simulink model "IEEE30_case"  (R2024b)
settings: Solver=FixedStepAuto  StartTime=0  StopTime=5  FixedStep=1e-7  RelTol=1e-3
values from neighbouring files (symbols this model uses):
  GFL_DFIG_7_C_bus = 0.08    [IEEE30_case_parameters.m]
  GFL_DFIG_7_D_mutual = 2.500000e+3    (= 2500)    [IEEE30_case_parameters.m]
  GFL_DFIG_7_f0 = 60    [IEEE30_case_parameters.m]
  GFL_DFIG_7_gPLLi = 3200    [IEEE30_case_parameters.m]
  GFL_DFIG_7_gPLLp = 650    [IEEE30_case_parameters.m]
  GFL_DFIG_7_H_WT = 0.4    [IEEE30_case_parameters.m]
  GFL_DFIG_7_Hg = 0.8    [IEEE30_case_parameters.m]
  GFL_DFIG_7_Igq_ref = 0    [IEEE30_case_parameters.m]
  GFL_DFIG_7_Ird_ref = 704.45696    [IEEE30_case_parameters.m]
  GFL_DFIG_7_KI_V = -300000    [IEEE30_case_parameters.m]
  GFL_DFIG_7_KP_V = -1000    [IEEE30_case_parameters.m]
  GFL_DFIG_7_Ksh = 1.254300e+4    (= 12543)    [IEEE30_case_parameters.m]
  GFL_DFIG_7_Lg = 0.000483    [IEEE30_case_parameters.m]
  GFL_DFIG_7_Lm_pu = 4    [IEEE30_case_parameters.m]
  GFL_DFIG_7_N = 100    [IEEE30_case_parameters.m]
  GFL_DFIG_7_p = 2    [IEEE30_case_parameters.m]
  GFL_DFIG_7_Pitch = 0    [IEEE30_case_parameters.m]
  GFL_DFIG_7_R = 44    [IEEE30_case_parameters.m]
  GFL_DFIG_7_Rg = 2.000000e-5    (= 2e-05)    [IEEE30_case_parameters.m]
  GFL_DFIG_7_rho = 1.225    [IEEE30_case_parameters.m]
  GFL_DFIG_7_rPLLi = 4500    [IEEE30_case_parameters.m]
  GFL_DFIG_7_rPLLp = 620    [IEEE30_case_parameters.m]
  GFL_DFIG_7_Rs_pu = 0.011    [IEEE30_case_parameters.m]
  GFL_DFIG_7_Sbase = 2.000000e+6    (= 2000000)    [IEEE30_case_parameters.m]
  GFL_DFIG_7_ugq_ref = 0    [IEEE30_case_parameters.m]
  GFL_DFIG_7_usd_ref = 0    [IEEE30_case_parameters.m]
  GFL_DFIG_7_Vbase = 690    [IEEE30_case_parameters.m]
  GFL_DFIG_7_Vdc_ref = 1200    [IEEE30_case_parameters.m]
  GFL_DFIG_7_wind = 12    [IEEE30_case_parameters.m]
  GFL_DFIG_7_wm_ref = 518.184209    [IEEE30_case_parameters.m]
  SG_D_13_D = 0.01056    [IEEE30_case_parameters.m]
  SG_D_13_EnableSaturation = 0    [IEEE30_case_parameters.m]
  SG_D_13_f0 = 60    [IEEE30_case_parameters.m]
  SG_D_13_H = 7.5    [IEEE30_case_parameters.m]
  SG_D_13_K_A = 20    [IEEE30_case_parameters.m]
  SG_D_13_K_E = 1.000000e+1    (= 10)    [IEEE30_case_parameters.m]
  SG_D_13_K_F = 2.363    [IEEE30_case_parameters.m]
  SG_D_13_K_s = 0.5    [IEEE30_case_parameters.m]
  SG_D_13_R_a = 0.001088    [IEEE30_case_parameters.m]
  SG_D_13_S_A = 1    [IEEE30_case_parameters.m]
  SG_D_13_S_B = 0.103    [IEEE30_case_parameters.m]
  SG_D_13_S_N = 10.659857    [IEEE30_case_parameters.m]
  SG_D_13_SpeedPara = 200    [IEEE30_case_parameters.m]
  SG_D_13_T_0 = 0.370163    [IEEE30_case_parameters.m]
  SG_D_13_T_1 = 0.3    [IEEE30_case_parameters.m]
  SG_D_13_T_2 = 0.05    [IEEE30_case_parameters.m]
  SG_D_13_T_3 = 0.02    [IEEE30_case_parameters.m]
  SG_D_13_T_4 = 0.005    [IEEE30_case_parameters.m]
  SG_D_13_T_A = 0.02    [IEEE30_case_parameters.m]
  SG_D_13_T_dd = 8.000000e+0    (= 8)    [IEEE30_case_parameters.m]
  SG_D_13_T_ddd = 0.04    [IEEE30_case_parameters.m]
  SG_D_13_T_E = 0.314    [IEEE30_case_parameters.m]
  SG_D_13_T_F = 0.35    [IEEE30_case_parameters.m]
  SG_D_13_T_qd = 0.8    [IEEE30_case_parameters.m]
  SG_D_13_T_qdd = 0.02    [IEEE30_case_parameters.m]
  SG_D_13_T_speed = 0.1    [IEEE30_case_parameters.m]
  SG_D_13_T_w = 0.5    [IEEE30_case_parameters.m]
  SG_D_13_V_ref = 1.696619    [IEEE30_case_parameters.m]
  SG_D_13_w_ref = 376.991118    [IEEE30_case_parameters.m]
  SG_D_13_x_d = 1.9    [IEEE30_case_parameters.m]
  SG_D_13_x_dd = 0.302    [IEEE30_case_parameters.m]
  SG_D_13_x_ddd = 0.204    [IEEE30_case_parameters.m]
  SG_D_13_x_l = 0.05    [IEEE30_case_parameters.m]
  SG_D_13_x_q = 1.3    [IEEE30_case_parameters.m]
  SG_D_13_x_qd = 0.5    [IEEE30_case_parameters.m]
  SG_D_13_x_qdd = 0.3    [IEEE30_case_parameters.m]
  SG_D_1_D = 0.01056    [IEEE30_case_parameters.m]
  SG_D_1_EnableSaturation = 0    [IEEE30_case_parameters.m]
  SG_D_1_f0 = 60    [IEEE30_case_parameters.m]
  SG_D_1_H = 7.5    [IEEE30_case_parameters.m]
  SG_D_1_K_A = 20    [IEEE30_case_parameters.m]
  SG_D_1_K_E = 1.000000e+1    (= 10)    [IEEE30_case_parameters.m]
  SG_D_1_K_F = 2.363    [IEEE30_case_parameters.m]
  SG_D_1_K_s = 0.5    [IEEE30_case_parameters.m]
  SG_D_1_R_a = 0.001088    [IEEE30_case_parameters.m]
  SG_D_1_S_A = 1    [IEEE30_case_parameters.m]
  SG_D_1_S_B = 0.103    [IEEE30_case_parameters.m]
  SG_D_1_S_N = 10.659857    [IEEE30_case_parameters.m]
  SG_D_1_SpeedPara = 200    [IEEE30_case_parameters.m]
  SG_D_1_T_0 = 0.259812    [IEEE30_case_parameters.m]
  SG_D_1_T_1 = 0.3    [IEEE30_case_parameters.m]
  SG_D_1_T_2 = 0.05    [IEEE30_case_parameters.m]
  SG_D_1_T_3 = 0.02    [IEEE30_case_parameters.m]
  SG_D_1_T_4 = 0.005    [IEEE30_case_parameters.m]
  SG_D_1_T_A = 0.02    [IEEE30_case_parameters.m]
  SG_D_1_T_dd = 8.000000e+0    (= 8)    [IEEE30_case_parameters.m]
  SG_D_1_T_ddd = 0.04    [IEEE30_case_parameters.m]
  SG_D_1_T_E = 0.314    [IEEE30_case_parameters.m]
  SG_D_1_T_F = 0.35    [IEEE30_case_parameters.m]
  SG_D_1_T_qd = 0.8    [IEEE30_case_parameters.m]
  SG_D_1_T_qdd = 0.02    [IEEE30_case_parameters.m]
  SG_D_1_T_speed = 0.1    [IEEE30_case_parameters.m]
  SG_D_1_T_w = 0.5    [IEEE30_case_parameters.m]
  SG_D_1_V_ref = 1.544107    [IEEE30_case_parameters.m]
  SG_D_1_w_ref = 376.991118    [IEEE30_case_parameters.m]
  SG_D_1_x_d = 1.9    [IEEE30_case_parameters.m]
  SG_D_1_x_dd = 0.302    [IEEE30_case_parameters.m]
  SG_D_1_x_ddd = 0.204    [IEEE30_case_parameters.m]
  SG_D_1_x_l = 0.05    [IEEE30_case_parameters.m]
  SG_D_1_x_q = 1.3    [IEEE30_case_parameters.m]
  SG_D_1_x_qd = 0.5    [IEEE30_case_parameters.m]
  SG_D_1_x_qdd = 0.3    [IEEE30_case_parameters.m]
  SG_D_22_D = 0.01056    [IEEE30_case_parameters.m]
  SG_D_22_EnableSaturation = 0    [IEEE30_case_parameters.m]
  SG_D_22_f0 = 60    [IEEE30_case_parameters.m]
  SG_D_22_H = 7.5    [IEEE30_case_parameters.m]
  SG_D_22_K_A = 20    [IEEE30_case_parameters.m]
  SG_D_22_K_E = 1.000000e+1    (= 10)    [IEEE30_case_parameters.m]
  SG_D_22_K_F = 2.363    [IEEE30_case_parameters.m]
  SG_D_22_K_s = 0.5    [IEEE30_case_parameters.m]
  SG_D_22_R_a = 0.001088    [IEEE30_case_parameters.m]
  SG_D_22_S_A = 1    [IEEE30_case_parameters.m]
  SG_D_22_S_B = 0.103    [IEEE30_case_parameters.m]
  SG_D_22_S_N = 10.659857    [IEEE30_case_parameters.m]
  SG_D_22_SpeedPara = 200    [IEEE30_case_parameters.m]
  SG_D_22_T_0 = 0.216121    [IEEE30_case_parameters.m]
  SG_D_22_T_1 = 0.3    [IEEE30_case_parameters.m]
  SG_D_22_T_2 = 0.05    [IEEE30_case_parameters.m]
  SG_D_22_T_3 = 0.02    [IEEE30_case_parameters.m]
  SG_D_22_T_4 = 0.005    [IEEE30_case_parameters.m]
  ... (+126 more)
(part 25 of 27)

== system IEEE30_case/SG_D_23/d_w_SG_D_23_block ==
  note: d_w_SG_D_23 in IEEE30_case
      | $\frac{2\,\pi \,T_{m,\mathrm{SG},D,23}\,f_{0}-D\,\left(w_{\mathrm{SG},D,23}-2\,\pi \,f_{0}\right)+2\,\pi \,f_{0}\,\left(\frac{\psi _{d,\mathrm{SG},D,23}\,\left(\psi _{q,\mathrm{SG},D,23}+\frac{\psi _{\mathrm{gq},\mathrm{SG},D,23}\,\left(x_{l}-x_{\mathrm{qdd}}\right)}{x_{l}-x_{\mathrm{qd}}}+\frac{\psi _{\mathrm{kq},\mathrm{SG},D,23}\,\left(x_{\mathrm{qd}}-x_{\mathrm{qdd}}\right)}{x_{l}-x_{\mathrm{qd}}}\right)}{x_{\mathrm{qdd}}}+\frac{\psi _{q,\mathrm{SG},D,23}\,\left(\frac{\psi _{\mathrm{1d},\mathrm{SG},D,23}\,\left(x_{\mathrm{dd}}-x_{\mathrm{ddd}}\right)}{x_{\mathrm{dd}}-x_{l}}-\psi _{d,\mathrm{SG},D,23}+\frac{\psi _{\mathrm{fd},\mathrm{SG},D,23}\,\left(x_{\mathrm{ddd}}-x_{l}\right)}{x_{\mathrm{dd}}-x_{l}}\right)}{x_{\mathrm{ddd}}}\right)}{2\,H}$
      | Automatically generated on 2025-11-01 18:37:27 .
  State_w_SG_D_23_a9c86 : Inport
  State_T_m_SG_D_23_67386 : Inport  Port=2
  State_psi_d_SG_D_23_cd292 : Inport  Port=3
  State_psi_gq_SG_D_23_30ca6 : Inport  Port=4
  State_psi_kq_SG_D_23_85da1 : Inport  Port=5
  State_psi_q_SG_D_23_ea802 : Inport  Port=6
  State_psi_q_SG_D_23_f4578 : Inport  Port=7
  State_psi_1d_SG_D_23_250d1 : Inport  Port=8
  State_psi_d_SG_D_23_77cdf : Inport  Port=9
  State_psi_fd_SG_D_23_fba26 : Inport  Port=10
  Add_34a9a : Sum
  Add_60312 : Sum
  Add_766b7 : Sum
  Add_877ab : Sum
  Add_a2dd3 : Sum
  Add_bf21f : Sum
  Add_cbb42 : Sum
  Add_ce37c : Sum
  Constant_-1_0529d : Constant  Value=-1
  Constant_-1_0665a : Constant  Value=-1
  Constant_-1_1274e : Constant  Value=-1
  Constant_-1_ae622 : Constant  Value=-1
  Constant_-1_bb572 : Constant  Value=-1
  Constant_-1_d880a : Constant  Value=-1
  Constant_-2.0_7e7ab : Constant  Value=-2.0
  Constant_2.0_0eeaf : Constant  Value=2.0
  Constant_2.0_8133d : Constant  Value=2.0
  Constant_2.0_86630 : Constant  Value=2.0
  Constant_D_d8423 : Constant  Value=D
  Constant_H_9e85c : Constant  Value=H
  Constant_f0_0164f : Constant  Value=f0
  Constant_f0_37545 : Constant  Value=f0
  Constant_f0_adf10 : Constant  Value=f0
  Constant_pi_89cee : Constant  Value=pi
  Constant_pi_ad3cb : Constant  Value=pi
  Constant_pi_f19cc : Constant  Value=pi
  Constant_x_dd_2dfc0 : Constant  Value=x_dd
  Constant_x_dd_49240 : Constant  Value=x_dd
  Constant_x_dd_d4555 : Constant  Value=x_dd
  Constant_x_ddd_5b4e5 : Constant  Value=x_ddd
  Constant_x_ddd_79b99 : Constant  Value=x_ddd
  Constant_x_ddd_80fee : Constant  Value=x_ddd
  Constant_x_l_03679 : Constant  Value=x_l
  Constant_x_l_34a4f : Constant  Value=x_l
  Constant_x_l_64425 : Constant  Value=x_l
  Constant_x_l_756be : Constant  Value=x_l
  Constant_x_l_91cbf : Constant  Value=x_l
  Constant_x_l_c7781 : Constant  Value=x_l
  Constant_x_qd_92bf4 : Constant  Value=x_qd
  Constant_x_qd_a2a78 : Constant  Value=x_qd
  Constant_x_qd_dda99 : Constant  Value=x_qd
  Constant_x_qdd_3c8ce : Constant  Value=x_qdd
  Constant_x_qdd_41b30 : Constant  Value=x_qdd
  Constant_x_qdd_81d75 : Constant  Value=x_qdd
  Divide_438bc : Product  Inputs=*/
  Divide_5c9e7 : Product  Inputs=*/
  Divide_64d37 : Product  Inputs=*/
  Divide_9ddc5 : Product  Inputs=*/
  Divide_c63d1 : Product  Inputs=*/
  Divide_dc8c0 : Product  Inputs=*/
  Divide_ea4bc : Product  Inputs=*/
  Product_024c1 : Product
  Product_072d4 : Product
  Product_1a3ea : Product
  Product_24bca : Product
  Product_392d6 : Product
  Product_3abdb : Product
  Product_4016c : Product
  Product_514ef : Product
  Product_55414 : Product
  Product_579b0 : Product
  Product_5df71 : Product
  Product_70ed9 : Product
  Product_75340 : Product
  Product_78ecf : Product
  Product_88dc9 : Product
  Product_8ee02 : Product
  Product_b37c8 : Product
  Product_c9e22 : Product
  Product_d29a1 : Product
  Product_eba4f : Product
  Product_ec235 : Product
  Product_f29ae : Product
  Subtract_30638 : Sum  Inputs=+-
  Subtract_5bb39 : Sum  Inputs=+-
  Subtract_a0565 : Sum  Inputs=+-
  Subtract_cf16a : Sum  Inputs=+-
  Subtract_cf1ab : Sum  Inputs=+-
  Subtract_d4472 : Sum  Inputs=+-
  Subtract_e17ae : Sum  Inputs=+-
  Subtract_f98fa : Sum  Inputs=+-
  Blockout_d_w_SG_D_23_057d1 : Outport
  wires:
  Constant_x_qdd_3c8ce/1 -> Add_877ab/2
  Constant_-1_0529d/1 -> Product_eba4f/1
  Product_eba4f/1 -> Add_877ab/1
  Constant_x_l_03679/1 -> Product_eba4f/2
  Product_78ecf/1 -> Add_a2dd3/1
  Constant_-1_bb572/1 -> Product_78ecf/1
  Subtract_cf1ab/1 -> Product_024c1/2
  Constant_x_qd_dda99/1 -> Subtract_cf1ab/1
  Constant_x_l_756be/1 -> Product_78ecf/2
  Constant_D_d8423/1 -> Product_d29a1/2
  Constant_x_qdd_41b30/1 -> Subtract_cf1ab/2
  Product_392d6/1 -> Add_cbb42/1
  Constant_-1_ae622/1 -> Product_392d6/1
  Constant_x_ddd_80fee/1 -> Subtract_cf16a/2
  Constant_-1_d880a/1 -> Product_d29a1/1
  Subtract_30638/1 -> Divide_438bc/2
  Constant_x_l_64425/1 -> Product_392d6/2
  Constant_-1_0665a/1 -> Product_5df71/1
  State_psi_1d_SG_D_23_250d1/1 -> Product_5df71/2
  State_psi_q_SG_D_23_ea802/1 -> Add_ce37c/2
  Constant_x_dd_d4555/1 -> Subtract_cf16a/1
  Constant_x_l_c7781/1 -> Subtract_a0565/2
  Product_579b0/1 -> Divide_ea4bc/1
  State_psi_gq_SG_D_23_30ca6/1 -> Product_579b0/1
  Add_877ab/1 -> Product_579b0/2
  Constant_x_qd_a2a78/1 -> Add_a2dd3/2
  Product_024c1/1 -> Divide_64d37/1
  State_psi_kq_SG_D_23_85da1/1 -> Product_024c1/1
  Subtract_cf16a/1 -> Product_1a3ea/2
  Constant_x_qd_92bf4/1 -> Add_cbb42/2
  Product_5df71/1 -> Product_1a3ea/1
  Constant_x_dd_2dfc0/1 -> Subtract_30638/1
  State_w_SG_D_23_a9c86/1 -> Add_766b7/2
  Product_ec235/1 -> Product_c9e22/1
  Constant_x_l_91cbf/1 -> Subtract_30638/2
  Constant_-1_1274e/1 -> Product_ec235/1
  Subtract_d4472/1 -> Product_8ee02/2
  Constant_x_ddd_5b4e5/1 -> Subtract_d4472/1
  Constant_x_l_34a4f/1 -> Subtract_d4472/2
  Constant_-2.0_7e7ab/1 -> Product_70ed9/1
  Add_a2dd3/1 -> Divide_ea4bc/2
  Add_cbb42/1 -> Divide_64d37/2
  Product_1a3ea/1 -> Divide_438bc/1
  Constant_2.0_8133d/1 -> Product_4016c/1
  Product_8ee02/1 -> Divide_5c9e7/1
  State_psi_fd_SG_D_23_fba26/1 -> Product_8ee02/1
  Subtract_a0565/1 -> Divide_5c9e7/2
  Constant_x_dd_49240/1 -> Subtract_a0565/1
  Divide_ea4bc/1 -> Subtract_5bb39/1
  Divide_64d37/1 -> Subtract_5bb39/2
  Divide_438bc/1 -> Add_60312/1
  State_psi_d_SG_D_23_77cdf/1 -> Add_60312/2
  Constant_pi_ad3cb/1 -> Product_70ed9/2
  State_psi_d_SG_D_23_cd292/1 -> Product_ec235/2
  Subtract_5bb39/1 -> Add_ce37c/1
  Add_60312/1 -> Subtract_e17ae/1
  Divide_5c9e7/1 -> Subtract_e17ae/2
  Product_70ed9/1 -> Product_514ef/1
  Constant_f0_0164f/1 -> Product_514ef/2
  Constant_pi_f19cc/1 -> Product_4016c/2
  Add_ce37c/1 -> Product_c9e22/2
  State_psi_q_SG_D_23_f4578/1 -> Product_b37c8/1
  Subtract_e17ae/1 -> Product_b37c8/2
  Product_514ef/1 -> Add_766b7/1
  Product_4016c/1 -> Product_75340/1
  State_T_m_SG_D_23_67386/1 -> Product_75340/2
  Constant_2.0_86630/1 -> Product_88dc9/1
  Constant_pi_89cee/1 -> Product_88dc9/2
  Product_c9e22/1 -> Divide_9ddc5/1
  Constant_x_qdd_81d75/1 -> Divide_9ddc5/2
  Product_b37c8/1 -> Divide_c63d1/1
  Constant_x_ddd_79b99/1 -> Divide_c63d1/2
  Product_d29a1/1 -> Product_072d4/1
  Add_766b7/1 -> Product_072d4/2
  Product_75340/1 -> Product_24bca/1
  Constant_f0_37545/1 -> Product_24bca/2
  Product_88dc9/1 -> Product_55414/1
  Constant_f0_adf10/1 -> Product_55414/2
  Divide_9ddc5/1 -> Add_bf21f/1
  Divide_c63d1/1 -> Add_bf21f/2
  Product_072d4/1 -> Add_34a9a/1
  Product_24bca/1 -> Add_34a9a/2
  Product_55414/1 -> Product_f29ae/1
  Add_bf21f/1 -> Product_f29ae/2
  Add_34a9a/1 -> Subtract_f98fa/1
  Product_f29ae/1 -> Subtract_f98fa/2
  Constant_2.0_0eeaf/1 -> Product_3abdb/1
  Constant_H_9e85c/1 -> Product_3abdb/2
  Subtract_f98fa/1 -> Divide_dc8c0/1
  Product_3abdb/1 -> Divide_dc8c0/2
  Divide_dc8c0/1 -> Blockout_d_w_SG_D_23_057d1/1

== system IEEE30_case/SG_D_23/i_d_SG_D_23_block ==
  note: i_d_SG_D_23 in IEEE30_case
      | $\frac{\sin\left(\theta _{\mathrm{SG},D,23}\right)\,\left(\frac{\psi _{\mathrm{1d},\mathrm{SG},D,23}\,\left(x_{\mathrm{dd}}-x_{\mathrm{ddd}}\right)}{x_{\mathrm{dd}}-x_{l}}-\psi _{d,\mathrm{SG},D,23}+\frac{\psi _{\mathrm{fd},\mathrm{SG},D,23}\,\left(x_{\mathrm{ddd}}-x_{l}\right)}{x_{\mathrm{dd}}-x_{l}}\right)}{x_{\mathrm{ddd}}}-\frac{\cos\left(\theta _{\mathrm{SG},D,23}\right)\,\left(\psi _{q,\mathrm{SG},D,23}+\frac{\psi _{\mathrm{gq},\mathrm{SG},D,23}\,\left(x_{l}-x_{\mathrm{qdd}}\right)}{x_{l}-x_{\mathrm{qd}}}+\frac{\psi _{\mathrm{kq},\mathrm{SG},D,23}\,\left(x_{\mathrm{qd}}-x_{\mathrm{qdd}}\right)}{x_{l}-x_{\mathrm{qd}}}\right)}{x_{\mathrm{qdd}}}$
      | Automatically generated on 2025-11-01 18:37:45 .
  State_psi_gq_SG_D_23_8a76e : Inport
  State_psi_kq_SG_D_23_a0ec4 : Inport  Port=2
  State_psi_q_SG_D_23_9f429 : Inport  Port=3
  State_theta_SG_D_23_46601 : Inport  Port=4
  State_psi_1d_SG_D_23_7111a : Inport  Port=5
  State_psi_d_SG_D_23_079bd : Inport  Port=6
  State_psi_fd_SG_D_23_8232a : Inport  Port=7
  State_theta_SG_D_23_15384 : Inport  Port=8
  Add_99617 : Sum
  Add_de10d : Sum
  Add_ed57c : Sum
  Add_ee6b8 : Sum
  Add_f683e : Sum
  Constant_-1_312cc : Constant  Value=-1
  Constant_-1_34ed3 : Constant  Value=-1
  Constant_-1_50e02 : Constant  Value=-1
  Constant_-1_7dce9 : Constant  Value=-1
  Constant_-1_936aa : Constant  Value=-1
  Constant_x_dd_20a3c : Constant  Value=x_dd
  Constant_x_dd_90625 : Constant  Value=x_dd
  Constant_x_dd_ca463 : Constant  Value=x_dd
  Constant_x_ddd_32f6c : Constant  Value=x_ddd
  Constant_x_ddd_7f849 : Constant  Value=x_ddd
  Constant_x_ddd_81b41 : Constant  Value=x_ddd
  Constant_x_l_22fb0 : Constant  Value=x_l
  Constant_x_l_3e953 : Constant  Value=x_l
  Constant_x_l_a1a1b : Constant  Value=x_l
  Constant_x_l_adba4 : Constant  Value=x_l
  Constant_x_l_c18b0 : Constant  Value=x_l
  Constant_x_l_db77a : Constant  Value=x_l
  Constant_x_qd_42c43 : Constant  Value=x_qd
  Constant_x_qd_7ef8d : Constant  Value=x_qd
  Constant_x_qd_b32fb : Constant  Value=x_qd
  Constant_x_qdd_7adc2 : Constant  Value=x_qdd
  Constant_x_qdd_837f5 : Constant  Value=x_qdd
  Constant_x_qdd_d77aa : Constant  Value=x_qdd
  Divide_259dc : Product  Inputs=*/
  Divide_31088 : Product  Inputs=*/
  Divide_79f4f : Product  Inputs=*/
  Divide_8d708 : Product  Inputs=*/
  Divide_f1559 : Product  Inputs=*/
  Divide_f7422 : Product  Inputs=*/
  MathFunc_cos_3d1b4 : Trigonometry  Operator=cos
  MathFunc_sin_1f2ca : Trigonometry
  Product_08031 : Product
  Product_2355a : Product
  Product_27067 : Product
  Product_418f8 : Product
  Product_6afa1 : Product
  Product_76679 : Product
  Product_7783e : Product
  Product_addf1 : Product
  Product_dc801 : Product
  Product_e0db2 : Product
  Product_f83ce : Product
  Subtract_0158c : Sum  Inputs=+-
  Subtract_04828 : Sum  Inputs=+-
  Subtract_19bce : Sum  Inputs=+-
  Subtract_2e06c : Sum  Inputs=+-
  Subtract_400c8 : Sum  Inputs=+-
  Subtract_86aa4 : Sum  Inputs=+-
  Subtract_87269 : Sum  Inputs=+-
  Subtract_fd2e5 : Sum  Inputs=+-
  Blockout_i_d_SG_D_23_e5d44 : Outport
  wires:
  Product_addf1/1 -> Divide_f1559/1
  Constant_-1_312cc/1 -> Product_dc801/1
  Constant_x_qdd_d77aa/1 -> Add_f683e/2
  Divide_79f4f/1 -> Subtract_19bce/2
  Constant_-1_50e02/1 -> Product_f83ce/1
  Product_7783e/1 -> Divide_79f4f/1
  State_psi_fd_SG_D_23_8232a/1 -> Product_7783e/1
  Constant_x_l_22fb0/1 -> Product_f83ce/2
  Product_2355a/1 -> Product_76679/1
  Product_6afa1/1 -> Divide_8d708/1
  Constant_x_qdd_7adc2/1 -> Subtract_87269/2
  Divide_f7422/1 -> Subtract_04828/1
  Product_f83ce/1 -> Add_f683e/1
  Constant_-1_7dce9/1 -> Product_e0db2/1
  MathFunc_cos_3d1b4/1 -> Product_08031/2
  State_theta_SG_D_23_46601/1 -> MathFunc_cos_3d1b4/1
  Constant_x_l_adba4/1 -> Product_e0db2/2
  Constant_x_qd_b32fb/1 -> Subtract_87269/1
  Subtract_19bce/1 -> Product_addf1/1
  Add_ee6b8/1 -> Divide_8d708/2
  Constant_x_l_db77a/1 -> Product_dc801/2
  Add_de10d/1 -> Divide_259dc/2
  State_psi_gq_SG_D_23_8a76e/1 -> Product_6afa1/1
  Add_f683e/1 -> Product_6afa1/2
  Product_e0db2/1 -> Add_ee6b8/1
  Constant_x_qd_7ef8d/1 -> Add_ee6b8/2
  Constant_-1_936aa/1 -> Product_2355a/1
  State_psi_kq_SG_D_23_a0ec4/1 -> Product_27067/1
  Subtract_87269/1 -> Product_27067/2
  Product_dc801/1 -> Add_de10d/1
  Constant_x_qd_42c43/1 -> Add_de10d/2
  State_psi_1d_SG_D_23_7111a/1 -> Product_2355a/2
  Constant_x_ddd_7f849/1 -> Divide_f1559/2
  Constant_x_dd_ca463/1 -> Subtract_fd2e5/1
  Constant_x_ddd_81b41/1 -> Subtract_fd2e5/2
  Product_27067/1 -> Divide_259dc/1
  Add_99617/1 -> Product_418f8/2
  Subtract_fd2e5/1 -> Product_76679/2
  Constant_x_dd_20a3c/1 -> Subtract_2e06c/1
  Constant_x_l_a1a1b/1 -> Subtract_2e06c/2
  Subtract_400c8/1 -> Product_7783e/2
  Constant_x_ddd_32f6c/1 -> Subtract_400c8/1
  Constant_x_l_3e953/1 -> Subtract_400c8/2
  Divide_8d708/1 -> Subtract_0158c/1
  Divide_259dc/1 -> Subtract_0158c/2
  Product_08031/1 -> Divide_f7422/1
  Product_76679/1 -> Divide_31088/1
  Subtract_2e06c/1 -> Divide_31088/2
  Subtract_86aa4/1 -> Divide_79f4f/2
  Constant_x_dd_90625/1 -> Subtract_86aa4/1
  Constant_x_l_c18b0/1 -> Subtract_86aa4/2
  Subtract_0158c/1 -> Add_99617/1
  State_psi_q_SG_D_23_9f429/1 -> Add_99617/2
  Divide_31088/1 -> Add_ed57c/1
  State_psi_d_SG_D_23_079bd/1 -> Add_ed57c/2
  Constant_-1_34ed3/1 -> Product_418f8/1
  Add_ed57c/1 -> Subtract_19bce/1
  MathFunc_sin_1f2ca/1 -> Product_addf1/2
  State_theta_SG_D_23_15384/1 -> MathFunc_sin_1f2ca/1
  Subtract_04828/1 -> Blockout_i_d_SG_D_23_e5d44/1
  Constant_x_qdd_837f5/1 -> Divide_f7422/2
  Product_418f8/1 -> Product_08031/1
  Divide_f1559/1 -> Subtract_04828/2

== system IEEE30_case/SG_D_23/i_q_SG_D_23_block ==
  note: i_q_SG_D_23 in IEEE30_case
      | $-\frac{\sin\left(\theta _{\mathrm{SG},D,23}\right)\,\left(\psi _{q,\mathrm{SG},D,23}+\frac{\psi _{\mathrm{gq},\mathrm{SG},D,23}\,\left(x_{l}-x_{\mathrm{qdd}}\right)}{x_{l}-x_{\mathrm{qd}}}+\frac{\psi _{\mathrm{kq},\mathrm{SG},D,23}\,\left(x_{\mathrm{qd}}-x_{\mathrm{qdd}}\right)}{x_{l}-x_{\mathrm{qd}}}\right)}{x_{\mathrm{qdd}}}-\frac{\cos\left(\theta _{\mathrm{SG},D,23}\right)\,\left(\frac{\psi _{\mathrm{1d},\mathrm{SG},D,23}\,\left(x_{\mathrm{dd}}-x_{\mathrm{ddd}}\right)}{x_{\mathrm{dd}}-x_{l}}-\psi _{d,\mathrm{SG},D,23}+\frac{\psi _{\mathrm{fd},\mathrm{SG},D,23}\,\left(x_{\mathrm{ddd}}-x_{l}\right)}{x_{\mathrm{dd}}-x_{l}}\right)}{x_{\mathrm{ddd}}}$
      | Automatically generated on 2025-11-01 18:37:50 .
  State_psi_gq_SG_D_23_3b4c4 : Inport
  State_psi_kq_SG_D_23_d1d5c : Inport  Port=2
  State_psi_q_SG_D_23_c45ba : Inport  Port=3
  State_theta_SG_D_23_c31a3 : Inport  Port=4
  State_psi_1d_SG_D_23_19122 : Inport  Port=5
  State_psi_d_SG_D_23_577bb : Inport  Port=6
  State_psi_fd_SG_D_23_b9ece : Inport  Port=7
  State_theta_SG_D_23_c16ba : Inport  Port=8
  Add_40d8d : Sum
  Add_4ae2a : Sum
  Add_573c3 : Sum
  Add_6cdcb : Sum
  Add_cfaac : Sum
  Add_f2645 : Sum
  Constant_-1_58374 : Constant  Value=-1
  Constant_-1_5d3a0 : Constant  Value=-1
  Constant_-1_c6427 : Constant  Value=-1
  Constant_-1_c999f : Constant  Value=-1
  Constant_-1_e8bcc : Constant  Value=-1
  Constant_x_dd_a0767 : Constant  Value=x_dd
  Constant_x_dd_aad58 : Constant  Value=x_dd
  Constant_x_dd_b9b12 : Constant  Value=x_dd
  Constant_x_ddd_3afe5 : Constant  Value=x_ddd
  Constant_x_ddd_65fae : Constant  Value=x_ddd
  Constant_x_ddd_885b5 : Constant  Value=x_ddd
  Constant_x_l_20736 : Constant  Value=x_l
  Constant_x_l_2a9d6 : Constant  Value=x_l
  Constant_x_l_3a9f1 : Constant  Value=x_l
  Constant_x_l_72430 : Constant  Value=x_l
  Constant_x_l_c5284 : Constant  Value=x_l
  Constant_x_l_d083f : Constant  Value=x_l
  Constant_x_qd_355aa : Constant  Value=x_qd
  Constant_x_qd_52434 : Constant  Value=x_qd
  Constant_x_qd_d7bb4 : Constant  Value=x_qd
  Constant_x_qdd_01ebd : Constant  Value=x_qdd
  Constant_x_qdd_aa134 : Constant  Value=x_qdd
  Constant_x_qdd_f67ba : Constant  Value=x_qdd
  Divide_13908 : Product  Inputs=*/
  Divide_13ab8 : Product  Inputs=*/
  Divide_2d93d : Product  Inputs=*/
  Divide_30293 : Product  Inputs=*/
  Divide_59a04 : Product  Inputs=*/
  Divide_8c936 : Product  Inputs=*/
  MathFunc_cos_790f2 : Trigonometry  Operator=cos
  MathFunc_sin_f0776 : Trigonometry
  Product_0bb89 : Product
  Product_2ae1e : Product
  Product_6a635 : Product
  Product_76692 : Product
  Product_98dff : Product
  Product_b23ed : Product
  Product_c9e90 : Product
  Product_e90a6 : Product
  Product_f576e : Product
  Product_f7fec : Product
  Product_fcf6b : Product
  Subtract_0c11d : Sum  Inputs=+-
  Subtract_640c1 : Sum  Inputs=+-
  Subtract_94cc8 : Sum  Inputs=+-
  Subtract_ba012 : Sum  Inputs=+-
  Subtract_c2950 : Sum  Inputs=+-
  Subtract_d2e13 : Sum  Inputs=+-
  Subtract_e8b1e : Sum  Inputs=+-
  Blockout_i_q_SG_D_23_6ad1e : Outport
  wires:
  Constant_x_ddd_65fae/1 -> Subtract_e8b1e/2
  Constant_x_l_20736/1 -> Product_f576e/2
  Constant_-1_58374/1 -> Product_f576e/1
  Product_f576e/1 -> Add_4ae2a/1
  Product_76692/1 -> Product_98dff/1
  Constant_-1_c999f/1 -> Product_76692/1
  Constant_x_qdd_01ebd/1 -> Subtract_c2950/2
  Constant_x_qdd_f67ba/1 -> Add_4ae2a/2
  Constant_x_qdd_aa134/1 -> Divide_2d93d/2
  Product_b23ed/1 -> Add_6cdcb/1
  Constant_-1_5d3a0/1 -> Product_b23ed/1
  Add_cfaac/1 -> Blockout_i_q_SG_D_23_6ad1e/1
  Add_40d8d/1 -> Product_6a635/2
  Product_c9e90/1 -> Divide_13908/1
  Subtract_c2950/1 -> Product_e90a6/2
  Constant_x_qd_355aa/1 -> Subtract_c2950/1
  Constant_x_l_d083f/1 -> Product_b23ed/2
  Product_2ae1e/1 -> Divide_2d93d/1
  Product_fcf6b/1 -> Add_f2645/1
  Constant_-1_c6427/1 -> Product_fcf6b/1
  Constant_x_l_2a9d6/1 -> Product_fcf6b/2
  MathFunc_cos_790f2/1 -> Product_0bb89/2
  State_theta_SG_D_23_c16ba/1 -> MathFunc_cos_790f2/1
  State_psi_1d_SG_D_23_19122/1 -> Product_76692/2
  State_psi_gq_SG_D_23_3b4c4/1 -> Product_c9e90/1
  Constant_-1_e8bcc/1 -> Product_6a635/1
  Add_4ae2a/1 -> Product_c9e90/2
  MathFunc_sin_f0776/1 -> Product_2ae1e/2
  Constant_x_qd_d7bb4/1 -> Add_6cdcb/2
  Product_e90a6/1 -> Divide_13ab8/1
  State_psi_kq_SG_D_23_d1d5c/1 -> Product_e90a6/1
  Constant_x_qd_52434/1 -> Add_f2645/2
  Constant_x_l_72430/1 -> Subtract_d2e13/2
  Subtract_e8b1e/1 -> Product_98dff/2
  Constant_x_dd_a0767/1 -> Subtract_e8b1e/1
  Add_6cdcb/1 -> Divide_13908/2
  Add_f2645/1 -> Divide_13ab8/2
  Subtract_0c11d/1 -> Divide_59a04/2
  Constant_x_dd_aad58/1 -> Subtract_0c11d/1
  Constant_x_l_c5284/1 -> Subtract_0c11d/2
  Subtract_640c1/1 -> Product_f7fec/2
  Constant_x_ddd_3afe5/1 -> Subtract_640c1/1
  Constant_x_l_3a9f1/1 -> Subtract_640c1/2
  Divide_13908/1 -> Subtract_ba012/1
  Divide_13ab8/1 -> Subtract_ba012/2
  Product_98dff/1 -> Divide_59a04/1
  Product_f7fec/1 -> Divide_8c936/1
  State_psi_fd_SG_D_23_b9ece/1 -> Product_f7fec/1
  Subtract_d2e13/1 -> Divide_8c936/2
  Constant_x_dd_b9b12/1 -> Subtract_d2e13/1
  Subtract_ba012/1 -> Add_40d8d/1
  State_psi_q_SG_D_23_c45ba/1 -> Add_40d8d/2
  Divide_59a04/1 -> Add_573c3/1
  State_psi_d_SG_D_23_577bb/1 -> Add_573c3/2
  State_theta_SG_D_23_c31a3/1 -> MathFunc_sin_f0776/1
  Product_6a635/1 -> Product_2ae1e/1
  Add_573c3/1 -> Subtract_94cc8/1
  Divide_8c936/1 -> Subtract_94cc8/2
  Subtract_94cc8/1 -> Product_0bb89/1
  Product_0bb89/1 -> Divide_30293/1
  Constant_x_ddd_885b5/1 -> Divide_30293/2
  Divide_2d93d/1 -> Add_cfaac/1
  Divide_30293/1 -> Add_cfaac/2

== system IEEE30_case/SG_D_23/theta_SG_D_23_out_block ==
  note: theta_SG_D_23_out in IEEE30_case
      | $\theta _{\mathrm{SG},D,23}$
      | Automatically generated on 2025-11-01 18:37:55 .
  State_theta_SG_D_23_9d978 : Inport
  Blockout_theta_SG_D_23_out_f3dde : Outport
  wires:
  State_theta_SG_D_23_9d978/1 -> Blockout_theta_SG_D_23_out_f3dde/1

== system IEEE30_case/SG_D_23/w_SG_D_23_out_block ==
  note: w_SG_D_23_out in IEEE30_case
      | $w_{\mathrm{SG},D,23}$
      | Automatically generated on 2025-11-01 18:37:55 .
  State_w_SG_D_23_a1e59 : Inport
  Blockout_w_SG_D_23_out_6070a : Outport
  wires:
  State_w_SG_D_23_a1e59/1 -> Blockout_w_SG_D_23_out_6070a/1

== system IEEE30_case/SG_D_27/T_e_SG_D_27_block ==
  note: T_e_SG_D_27 in IEEE30_case
      | $-\frac{\psi _{d,\mathrm{SG},D,27}\,\left(\psi _{q,\mathrm{SG},D,27}+\frac{\psi _{\mathrm{gq},\mathrm{SG},D,27}\,\left(x_{l}-x_{\mathrm{qdd}}\right)}{x_{l}-x_{\mathrm{qd}}}+\frac{\psi _{\mathrm{kq},\mathrm{SG},D,27}\,\left(x_{\mathrm{qd}}-x_{\mathrm{qdd}}\right)}{x_{l}-x_{\mathrm{qd}}}\right)}{x_{\mathrm{qdd}}}-\frac{\psi _{q,\mathrm{SG},D,27}\,\left(\frac{\psi _{\mathrm{1d},\mathrm{SG},D,27}\,\left(x_{\mathrm{dd}}-x_{\mathrm{ddd}}\right)}{x_{\mathrm{dd}}-x_{l}}-\psi _{d,\mathrm{SG},D,27}+\frac{\psi _{\mathrm{fd},\mathrm{SG},D,27}\,\left(x_{\mathrm{ddd}}-x_{l}\right)}{x_{\mathrm{dd}}-x_{l}}\right)}{x_{\mathrm{ddd}}}$
      | Automatically generated on 2025-11-01 18:39:03 .
  State_psi_d_SG_D_27_aae51 : Inport
  State_psi_gq_SG_D_27_2222e : Inport  Port=2
  State_psi_kq_SG_D_27_9e25d : Inport  Port=3
  State_psi_q_SG_D_27_c3716 : Inport  Port=4
  State_psi_q_SG_D_27_f2155 : Inport  Port=5
  State_psi_1d_SG_D_27_3beb4 : Inport  Port=6
  State_psi_d_SG_D_27_1e6e0 : Inport  Port=7
  State_psi_fd_SG_D_27_93998 : Inport  Port=8
  Add_58dd4 : Sum
  Add_62b21 : Sum
  Add_6e466 : Sum
  Add_899d1 : Sum
  Add_bf566 : Sum
  Add_cc99a : Sum
  Constant_-1_0339b : Constant  Value=-1
  Constant_-1_76629 : Constant  Value=-1
  Constant_-1_a29db : Constant  Value=-1
  Constant_-1_aebb2 : Constant  Value=-1
  Constant_-1_e217e : Constant  Value=-1
  Constant_x_dd_1da9f : Constant  Value=x_dd
  Constant_x_dd_4bd6a : Constant  Value=x_dd
  Constant_x_dd_a2584 : Constant  Value=x_dd
  Constant_x_ddd_0b1a3 : Constant  Value=x_ddd
  Constant_x_ddd_d560c : Constant  Value=x_ddd
  Constant_x_ddd_e9a7e : Constant  Value=x_ddd
  Constant_x_l_0705f : Constant  Value=x_l
  Constant_x_l_1c38b : Constant  Value=x_l
  Constant_x_l_37715 : Constant  Value=x_l
  Constant_x_l_4b2a4 : Constant  Value=x_l
  Constant_x_l_7000a : Constant  Value=x_l
  Constant_x_l_7b0ba : Constant  Value=x_l
  Constant_x_qd_1bbcc : Constant  Value=x_qd
  Constant_x_qd_51226 : Constant  Value=x_qd
  Constant_x_qd_613e8 : Constant  Value=x_qd
  Constant_x_qdd_0cc21 : Constant  Value=x_qdd
  Constant_x_qdd_249d0 : Constant  Value=x_qdd
  Constant_x_qdd_3834a : Constant  Value=x_qdd
  Divide_62fff : Product  Inputs=*/
  Divide_676ea : Product  Inputs=*/
  Divide_b3eff : Product  Inputs=*/
  Divide_b4cfc : Product  Inputs=*/
  Divide_c55f5 : Product  Inputs=*/
  Divide_dca8c : Product  Inputs=*/
  Product_27d11 : Product
  Product_371ec : Product
  Product_676e4 : Product
  Product_86347 : Product
  Product_8cf2a : Product
  Product_a3725 : Product
  Product_aa5a8 : Product
  Product_b0103 : Product
  Product_b28be : Product
  Product_c1c10 : Product
  Product_cc939 : Product
  Subtract_0b899 : Sum  Inputs=+-
  Subtract_12b2d : Sum  Inputs=+-
  Subtract_5e278 : Sum  Inputs=+-
  Subtract_96f38 : Sum  Inputs=+-
  Subtract_c8542 : Sum  Inputs=+-
  Subtract_e2867 : Sum  Inputs=+-
  Subtract_ee4c3 : Sum  Inputs=+-
  Blockout_T_e_SG_D_27_0afee : Outport
  wires:
  Divide_62fff/1 -> Add_cc99a/1
  Product_cc939/1 -> Divide_676ea/1
  Constant_-1_e217e/1 -> Product_86347/1
  Constant_x_qdd_0cc21/1 -> Add_bf566/2
  Subtract_96f38/1 -> Product_c1c10/2
  Subtract_5e278/1 -> Product_cc939/2
  Constant_x_l_0705f/1 -> Product_86347/2
  State_psi_1d_SG_D_27_3beb4/1 -> Product_371ec/2
  Product_86347/1 -> Add_bf566/1
  Add_6e466/1 -> Blockout_T_e_SG_D_27_0afee/1
  Product_c1c10/1 -> Divide_dca8c/1
  Constant_-1_76629/1 -> Product_a3725/1
  Add_cc99a/1 -> Subtract_96f38/1
  Constant_x_qd_1bbcc/1 -> Subtract_5e278/1
  Product_a3725/1 -> Add_899d1/1
  Constant_x_l_4b2a4/1 -> Product_a3725/2
  Product_b0103/1 -> Product_8cf2a/1
  Constant_x_qdd_249d0/1 -> Subtract_5e278/2
  Constant_-1_a29db/1 -> Product_aa5a8/1
  Constant_x_l_7b0ba/1 -> Product_aa5a8/2
  Constant_x_ddd_e9a7e/1 -> Divide_dca8c/2
  Constant_-1_aebb2/1 -> Product_371ec/1
  Constant_x_dd_1da9f/1 -> Subtract_c8542/1
  Constant_x_ddd_0b1a3/1 -> Subtract_c8542/2
  State_psi_gq_SG_D_27_2222e/1 -> Product_b28be/1
  Subtract_12b2d/1 -> Divide_b4cfc/2
  Add_bf566/1 -> Product_b28be/2
  Constant_x_qd_51226/1 -> Add_899d1/2
  Product_27d11/1 -> Divide_62fff/1
  State_psi_kq_SG_D_27_9e25d/1 -> Product_cc939/1
  Product_aa5a8/1 -> Add_62b21/1
  Constant_x_qd_613e8/1 -> Add_62b21/2
  Constant_x_l_37715/1 -> Subtract_12b2d/2
  Product_371ec/1 -> Product_27d11/1
  Subtract_c8542/1 -> Product_27d11/2
  Constant_x_dd_4bd6a/1 -> Subtract_e2867/1
  Constant_-1_0339b/1 -> Product_b0103/1
  Constant_x_l_1c38b/1 -> Subtract_e2867/2
  Constant_x_ddd_d560c/1 -> Subtract_0b899/1
  Divide_b3eff/1 -> Add_6e466/1
  Constant_x_l_7000a/1 -> Subtract_0b899/2
  State_psi_q_SG_D_27_f2155/1 -> Product_c1c10/1
  Product_b28be/1 -> Divide_c55f5/1
  Add_899d1/1 -> Divide_c55f5/2
  Add_62b21/1 -> Divide_676ea/2
  Subtract_e2867/1 -> Divide_62fff/2
  Add_58dd4/1 -> Product_8cf2a/2
  State_psi_fd_SG_D_27_93998/1 -> Product_676e4/1
  Subtract_0b899/1 -> Product_676e4/2
  Constant_x_dd_a2584/1 -> Subtract_12b2d/1
  Divide_c55f5/1 -> Subtract_ee4c3/1
  Divide_dca8c/1 -> Add_6e466/2
  Divide_676ea/1 -> Subtract_ee4c3/2
  State_psi_d_SG_D_27_1e6e0/1 -> Add_cc99a/2
  Product_676e4/1 -> Divide_b4cfc/1
  Product_8cf2a/1 -> Divide_b3eff/1
  State_psi_d_SG_D_27_aae51/1 -> Product_b0103/2
  Subtract_ee4c3/1 -> Add_58dd4/1
  State_psi_q_SG_D_27_c3716/1 -> Add_58dd4/2
  Divide_b4cfc/1 -> Subtract_96f38/2
  Constant_x_qdd_3834a/1 -> Divide_b3eff/2

== system IEEE30_case/SG_D_27/d_E_fd_SG_D_27_block ==
  note: d_E_fd_SG_D_27 in IEEE30_case
      | $\frac{V_{f,\mathrm{SG},D,27}-E_{\mathrm{fd},\mathrm{SG},D,27}\,K_{E}}{T_{E}}$
      | Automatically generated on 2025-11-01 18:38:46 .
  State_E_fd_SG_D_27_823cb : Inport
  State_V_f_SG_D_27_0da35 : Inport  Port=2
  Add_48682 : Sum
  Constant_-1_b8de2 : Constant  Value=-1
  Constant_K_E_0e495 : Constant  Value=K_E
  Constant_T_E_fb76b : Constant  Value=T_E
  Divide_654ca : Product  Inputs=*/
  Product_5b916 : Product
  Product_f51cd : Product
  Blockout_d_E_fd_SG_D_27_b9ef8 : Outport
  wires:
  State_E_fd_SG_D_27_823cb/1 -> Product_5b916/2
  Constant_-1_b8de2/1 -> Product_5b916/1
  Constant_K_E_0e495/1 -> Product_f51cd/2
  Product_5b916/1 -> Product_f51cd/1
  Add_48682/1 -> Divide_654ca/1
  Divide_654ca/1 -> Blockout_d_E_fd_SG_D_27_b9ef8/1
  Product_f51cd/1 -> Add_48682/1
  State_V_f_SG_D_27_0da35/1 -> Add_48682/2
  Constant_T_E_fb76b/1 -> Divide_654ca/2

== system IEEE30_case/SG_D_27/d_Px_1_SG_D_27_block ==
  note: d_Px_1_SG_D_27 in IEEE30_case
      | $\frac{w_{\mathrm{SG},D,27}-2\,\pi \,f_{0}}{T_{w}}-\frac{\mathrm{Px}_{1,\mathrm{SG},D,27}}{T_{w}}$
      | Automatically generated on 2025-11-01 18:38:47 .
  State_Px_1_SG_D_27_e0716 : Inport
  State_w_SG_D_27_cf173 : Inport  Port=2
  Add_22452 : Sum
  Add_afb5d : Sum
  Constant_-1_262bf : Constant  Value=-1
  Constant_-2.0_7f85f : Constant  Value=-2.0
  Constant_T_w_1847e : Constant  Value=T_w
  Constant_T_w_34261 : Constant  Value=T_w
  Constant_f0_c26b3 : Constant  Value=f0
  Constant_pi_44e21 : Constant  Value=pi
  Divide_7c605 : Product  Inputs=*/
  Divide_a225a : Product  Inputs=*/
  Product_103b8 : Product
  Product_12144 : Product
  Product_362eb : Product
  Blockout_d_Px_1_SG_D_27_439b8 : Outport
  wires:
  Constant_-2.0_7f85f/1 -> Product_362eb/1
  Product_103b8/1 -> Add_22452/1
  Constant_pi_44e21/1 -> Product_362eb/2
  Constant_f0_c26b3/1 -> Product_103b8/2
  Product_362eb/1 -> Product_103b8/1
  State_w_SG_D_27_cf173/1 -> Add_22452/2
  Constant_-1_262bf/1 -> Product_12144/1
  State_Px_1_SG_D_27_e0716/1 -> Product_12144/2
  Product_12144/1 -> Divide_7c605/1
  Constant_T_w_34261/1 -> Divide_7c605/2
  Add_22452/1 -> Divide_a225a/1
  Constant_T_w_1847e/1 -> Divide_a225a/2
  Divide_7c605/1 -> Add_afb5d/1
  Divide_a225a/1 -> Add_afb5d/2
  Add_afb5d/1 -> Blockout_d_Px_1_SG_D_27_439b8/1

== system IEEE30_case/SG_D_27/d_Px_2_SG_D_27_block ==
  note: d_Px_2_SG_D_27 in IEEE30_case
      | $\frac{\mathrm{Px}_{1,\mathrm{SG},D,27}-T_{2}\,\left(\frac{\mathrm{Px}_{1,\mathrm{SG},D,27}}{T_{w}}-\frac{w_{\mathrm{SG},D,27}-2\,\pi \,f_{0}}{T_{w}}\right)}{T_{1}}-\frac{\mathrm{Px}_{2,\mathrm{SG},D,27}}{T_{1}}$
      | Automatically generated on 2025-11-01 18:38:49 .
  State_Px_2_SG_D_27_373db : Inport
  State_Px_1_SG_D_27_13dd5 : Inport  Port=2
  State_Px_1_SG_D_27_849c9 : Inport  Port=3
  State_w_SG_D_27_5c50a : Inport  Port=4
  Add_46263 : Sum
  Add_47a2b : Sum
  Add_59103 : Sum
  Add_94a02 : Sum
  Constant_-1_08b4f : Constant  Value=-1
  Constant_-1_ffc91 : Constant  Value=-1
  Constant_-2.0_6cb4a : Constant  Value=-2.0
  Constant_T_1_09a42 : Constant  Value=T_1
  Constant_T_1_7d634 : Constant  Value=T_1
  Constant_T_2_00f19 : Constant  Value=T_2
  Constant_T_w_9b1ed : Constant  Value=T_w
  Constant_T_w_fb965 : Constant  Value=T_w
  Constant_f0_06efd : Constant  Value=f0
  Constant_pi_67fa7 : Constant  Value=pi
  Divide_631f6 : Product  Inputs=*/
  Divide_84317 : Product  Inputs=*/
  Divide_cc441 : Product  Inputs=*/
  Divide_f707a : Product  Inputs=*/
  Product_14717 : Product
  Product_26973 : Product
  Product_64866 : Product
  Product_bd34f : Product
  Product_cc03e : Product
  Blockout_d_Px_2_SG_D_27_55afa : Outport
  wires:
  Divide_631f6/1 -> Add_47a2b/1
  State_Px_1_SG_D_27_849c9/1 -> Product_bd34f/2
  Constant_f0_06efd/1 -> Product_cc03e/2
  Constant_-2.0_6cb4a/1 -> Product_26973/1
  Product_26973/1 -> Product_cc03e/1
  Product_cc03e/1 -> Add_46263/1
  Constant_pi_67fa7/1 -> Product_26973/2
  Product_bd34f/1 -> Divide_631f6/1
  Constant_-1_08b4f/1 -> Product_bd34f/1
  Divide_84317/1 -> Add_94a02/1
  State_w_SG_D_27_5c50a/1 -> Add_46263/2
  Product_64866/1 -> Add_59103/2
  Constant_T_2_00f19/1 -> Product_64866/1
  Constant_T_w_fb965/1 -> Divide_631f6/2
  Add_46263/1 -> Divide_f707a/1
  Constant_T_w_9b1ed/1 -> Divide_f707a/2
  Divide_f707a/1 -> Add_47a2b/2
  Add_47a2b/1 -> Product_64866/2
  Constant_-1_ffc91/1 -> Product_14717/1
  State_Px_2_SG_D_27_373db/1 -> Product_14717/2
  Add_59103/1 -> Divide_cc441/1
  State_Px_1_SG_D_27_13dd5/1 -> Add_59103/1
  Product_14717/1 -> Divide_84317/1
  Constant_T_1_09a42/1 -> Divide_84317/2
  Constant_T_1_7d634/1 -> Divide_cc441/2
  Divide_cc441/1 -> Add_94a02/2
  Add_94a02/1 -> Blockout_d_Px_2_SG_D_27_55afa/1

== system IEEE30_case/SG_D_27/d_Px_3_SG_D_27_block ==
  note: d_Px_3_SG_D_27 in IEEE30_case
      | $\frac{\mathrm{Px}_{2,\mathrm{SG},D,27}+T_{4}\,\left(\frac{\mathrm{Px}_{1,\mathrm{SG},D,27}-T_{2}\,\left(\frac{\mathrm{Px}_{1,\mathrm{SG},D,27}}{T_{w}}-\frac{w_{\mathrm{SG},D,27}-2\,\pi \,f_{0}}{T_{w}}\right)}{T_{1}}-\frac{\mathrm{Px}_{2,\mathrm{SG},D,27}}{T_{1}}\right)}{T_{3}}-\frac{\mathrm{Px}_{3,\mathrm{SG},D,27}}{T_{3}}$
      | Automatically generated on 2025-11-01 18:38:51 .
  State_Px_3_SG_D_27_7eb86 : Inport
  State_Px_2_SG_D_27_7e14b : Inport  Port=2
  State_Px_2_SG_D_27_a8fab : Inport  Port=3
  State_Px_1_SG_D_27_bbb95 : Inport  Port=4
  State_Px_1_SG_D_27_e5cc3 : Inport  Port=5
  State_w_SG_D_27_62987 : Inport  Port=6
  Add_51e20 : Sum
  Add_a4816 : Sum
  Add_b8d7b : Sum
  Add_b9876 : Sum
  Add_f9525 : Sum
  Add_fe742 : Sum
  Constant_-1_1cd6b : Constant  Value=-1
  Constant_-1_a4f86 : Constant  Value=-1
  Constant_-1_ce658 : Constant  Value=-1
  Constant_-2.0_efe86 : Constant  Value=-2.0
  Constant_T_1_24092 : Constant  Value=T_1
  Constant_T_1_95641 : Constant  Value=T_1
  Constant_T_2_d9632 : Constant  Value=T_2
  Constant_T_3_4372a : Constant  Value=T_3
  Constant_T_3_6a972 : Constant  Value=T_3
  Constant_T_4_5ce1d : Constant  Value=T_4
  Constant_T_w_5790c : Constant  Value=T_w
  Constant_T_w_d4fd1 : Constant  Value=T_w
  Constant_f0_24778 : Constant  Value=f0
  Constant_pi_ac239 : Constant  Value=pi
  Divide_17362 : Product  Inputs=*/
  Divide_22c96 : Product  Inputs=*/
  Divide_87250 : Product  Inputs=*/
  Divide_95976 : Product  Inputs=*/
  Divide_e705a : Product  Inputs=*/
  Divide_ea44b : Product  Inputs=*/
  Product_60ff9 : Product
  Product_6fd5f : Product
  Product_9425d : Product
  Product_bdd3c : Product
  Product_d3967 : Product
  Product_e0880 : Product
  Product_faa19 : Product
  Blockout_d_Px_3_SG_D_27_484b3 : Outport
  wires:
  State_Px_1_SG_D_27_e5cc3/1 -> Product_bdd3c/2
  Constant_-2.0_efe86/1 -> Product_d3967/1
  Product_d3967/1 -> Product_faa19/1
  Constant_f0_24778/1 -> Product_faa19/2
  Constant_pi_ac239/1 -> Product_d3967/2
  Product_faa19/1 -> Add_a4816/1
  Product_bdd3c/1 -> Divide_87250/1
  Constant_-1_a4f86/1 -> Product_bdd3c/1
  Divide_e705a/1 -> Add_51e20/2
  State_w_SG_D_27_62987/1 -> Add_a4816/2
  Constant_T_w_d4fd1/1 -> Divide_87250/2
  Constant_T_w_5790c/1 -> Divide_e705a/2
  Add_a4816/1 -> Divide_e705a/1
  Divide_87250/1 -> Add_51e20/1
  Constant_T_3_6a972/1 -> Divide_17362/2
  Product_e0880/1 -> Add_b8d7b/2
  Constant_T_2_d9632/1 -> Product_e0880/1
  Add_51e20/1 -> Product_e0880/2
  Product_6fd5f/1 -> Divide_95976/1
  Constant_-1_ce658/1 -> Product_6fd5f/1
  State_Px_2_SG_D_27_a8fab/1 -> Product_6fd5f/2
  Add_fe742/1 -> Blockout_d_Px_3_SG_D_27_484b3/1
  Add_b8d7b/1 -> Divide_22c96/1
  State_Px_1_SG_D_27_bbb95/1 -> Add_b8d7b/1
  Divide_22c96/1 -> Add_b9876/2
  Constant_T_1_24092/1 -> Divide_95976/2
  Constant_T_1_95641/1 -> Divide_22c96/2
  Divide_95976/1 -> Add_b9876/1
  Constant_T_4_5ce1d/1 -> Product_60ff9/1
  Divide_17362/1 -> Add_fe742/1
  Add_b9876/1 -> Product_60ff9/2
  Constant_-1_1cd6b/1 -> Product_9425d/1
  State_Px_3_SG_D_27_7eb86/1 -> Product_9425d/2
  State_Px_2_SG_D_27_7e14b/1 -> Add_f9525/1
  Product_60ff9/1 -> Add_f9525/2
  Product_9425d/1 -> Divide_17362/1
  Add_f9525/1 -> Divide_ea44b/1
  Constant_T_3_4372a/1 -> Divide_ea44b/2
  Divide_ea44b/1 -> Add_fe742/2

== system IEEE30_case/SG_D_27/d_R_f_SG_D_27_block ==
  note: d_R_f_SG_D_27 in IEEE30_case
      | $-\frac{R_{f,\mathrm{SG},D,27}-\frac{E_{\mathrm{fd},\mathrm{SG},D,27}\,K_{F}}{T_{F}}}{T_{F}}$
      | Automatically generated on 2025-11-01 18:38:45 .
  State_E_fd_SG_D_27_e31da : Inport
  State_R_f_SG_D_27_31c67 : Inport  Port=2
  Constant_K_F_92426 : Constant  Value=K_F
  Constant_T_F_485ee : Constant  Value=T_F
  Constant_T_F_e86ec : Constant  Value=T_F
  Divide_ba574 : Product  Inputs=*/
  Divide_f5385 : Product  Inputs=*/
  Product_969c3 : Product
  Subtract_662be : Sum  Inputs=+-
  Blockout_d_R_f_SG_D_27_9dd2c : Outport
  wires:
  State_E_fd_SG_D_27_e31da/1 -> Product_969c3/1
  Constant_K_F_92426/1 -> Product_969c3/2
  Product_969c3/1 -> Divide_ba574/1
  Constant_T_F_485ee/1 -> Divide_f5385/2
  Divide_ba574/1 -> Subtract_662be/1
  Constant_T_F_e86ec/1 -> Divide_ba574/2
  State_R_f_SG_D_27_31c67/1 -> Subtract_662be/2
  Subtract_662be/1 -> Divide_f5385/1
  Divide_f5385/1 -> Blockout_d_R_f_SG_D_27_9dd2c/1

== system IEEE30_case/SG_D_27/d_T_m_SG_D_27_block ==
  note: d_T_m_SG_D_27 in IEEE30_case
      | $-\frac{T_{m,\mathrm{SG},D,27}-T_{0}+\frac{\mathrm{SpeedPara}\,\left(w_{\mathrm{SG},D,27}-w_{\mathrm{ref}}\right)}{2\,f_{0}\,\pi }}{T_{\mathrm{speed}}}$
      | Automatically generated on 2025-11-01 18:38:35 .
  State_w_SG_D_27_b53f8 : Inport
  State_T_m_SG_D_27_0f28d : Inport  Port=2
  Add_3d292 : Sum
  Add_c372f : Sum
  Constant_-1_d630d : Constant  Value=-1
  Constant_2.0_7fd06 : Constant  Value=2.0
  Constant_SpeedPara_318a4 : Constant  Value=SpeedPara
  Constant_T_0_0bf0c : Constant  Value=T_0
  Constant_T_speed_ff7c8 : Constant  Value=T_speed
  Constant_f0_76fab : Constant  Value=f0
  Constant_pi_f4ad0 : Constant  Value=pi
  Constant_w_ref_aab4f : Constant  Value=w_ref
  Divide_81ede : Product  Inputs=*/
  Divide_fc673 : Product  Inputs=*/
  Product_39904 : Product
  Product_878d5 : Product
  Product_a689f : Product
  Product_acb43 : Product
  Subtract_36d64 : Sum  Inputs=+-
  Blockout_d_T_m_SG_D_27_75196 : Outport
  wires:
  State_w_SG_D_27_b53f8/1 -> Product_878d5/2
  Constant_-1_d630d/1 -> Product_878d5/1
  Product_878d5/1 -> Add_3d292/1
  Constant_SpeedPara_318a4/1 -> Product_acb43/1
  Constant_w_ref_aab4f/1 -> Add_3d292/2
  Constant_2.0_7fd06/1 -> Product_a689f/1
  Add_3d292/1 -> Product_acb43/2
  Constant_pi_f4ad0/1 -> Product_a689f/2
  Product_a689f/1 -> Product_39904/1
  Constant_f0_76fab/1 -> Product_39904/2
  Product_39904/1 -> Divide_fc673/2
  Product_acb43/1 -> Divide_fc673/1
  Divide_fc673/1 -> Add_c372f/1
  Constant_T_0_0bf0c/1 -> Add_c372f/2
  State_T_m_SG_D_27_0f28d/1 -> Subtract_36d64/2
  Add_c372f/1 -> Subtract_36d64/1
  Subtract_36d64/1 -> Divide_81ede/1
  Constant_T_speed_ff7c8/1 -> Divide_81ede/2
  Divide_81ede/1 -> Blockout_d_T_m_SG_D_27_75196/1
